simulink model "BESSINDPROJ"  (R2023b)
settings: Solver=VariableStepAuto  StartTime=0.0  StopTime=0.8  RelTol=1e-3
undefined symbols (not defined in the file): Ion, Lithium, Pnom1, Ts_Control, Ts_Power, Vnom_prim
libraries: spsSeriesRLCBranchLib x8, slpidlib x4, spsVoltageMeasurementLib x4, spsPowerLib x3, spsMeanLib x2, spsPWMGeneratorDCDCLib x2, spsCurrentMeasurementLib x2, spsMosfetLib x2, spsMultimeterLib x2, spsBatteryLib x1, spsSeriesRLCLoadLib x1, spsFundamentalPLLDrivenLib x1
settings Model: Creator=michelkhalil  LastModifiedBy=michelkhalil

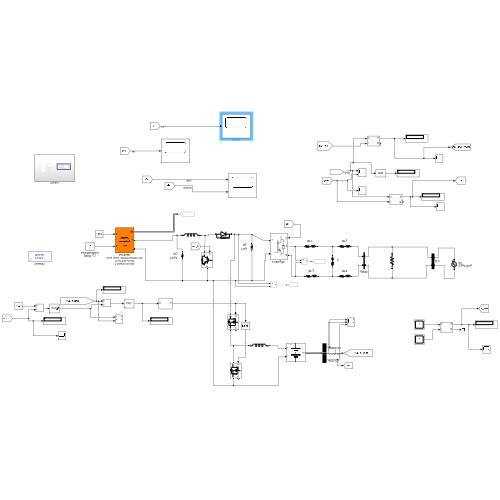
[thumbnail: Simulink's stored preview of the top-level diagram]
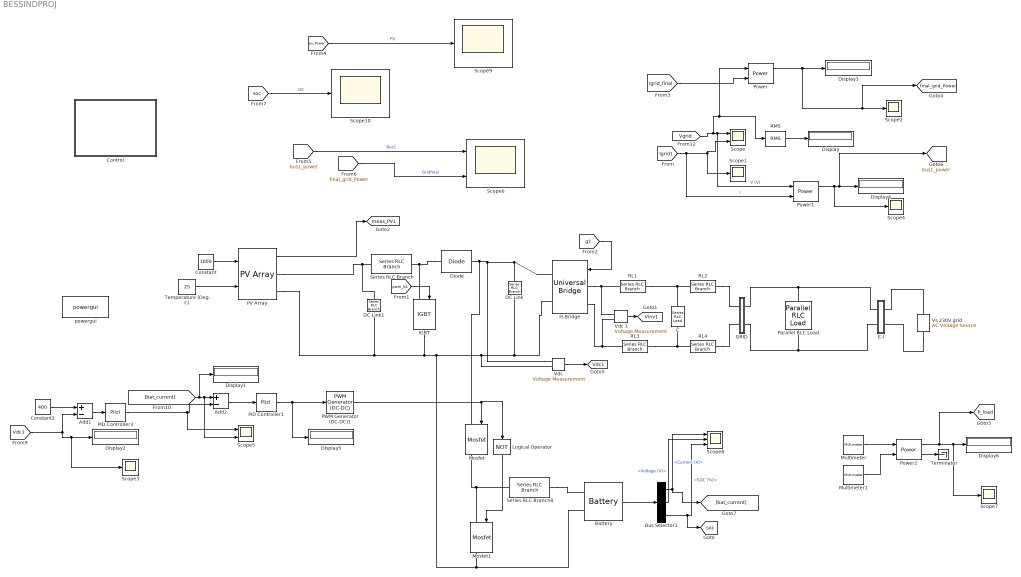
== system BESSINDPROJ ==
  Add1 : Sum  Inputs=+-
  Add2 : Sum  Inputs=+-
  Battery : spsBatteryLib/Battery  BatType=Lithium-Ion  ShowTempParam=off  ThermalPreset=no  ShowAgeParam=off  NomV=96  NomQ=50  SOC=60  Batt_Tr=30  PresetModel=on  MaxQ=50  MinV=72  FullV=111.7428  Dis_rate=21.7391  R=0.0192  Normal_OP=45.2174  expZone="[103.717      2.456522]"  current=[6.5 13 32.5]  Units=Time  Tci=20  NomT=20  T2=-30  MaxQ2=4.8  FullV2=7.1  Normal_OP2=5.655  expZone2="[6.58           1]"  Rca=0.6  ti=2000  Dp=0  Neq0=0  Tsim=1e6  Ta1=25  Qeol=5.4*0.9  Reol=0.013333*1.2  Char_age=[2.3478, 3]  Dis_age=[2.3478, 10]  N1=1500  N2=10500  N3=1000  N4=1400  Ta2=45  N5=950
  Bus Selector1 : BusSelector  OutputSignals=Current (A),Voltage (V),SOC (%)
  C : spsSeriesRLCLoadLib/Series RLC Load  LConnTagsString=a  RConnTagsString=__new0  NominalVoltage=240  NominalFrequency=50  ActivePower=10.5  InductivePower=0  CapacitivePower=525  Setx0=off  InitialVoltage=0  SetiL0=off  InitialCurrent=0  Measurements=None  LoadType=constant Z
  Constant : Constant  Value=1000
  Constant2 : Constant  Value=400
  Control : Subsystem
  DC Link : spsSeriesRLCBranchLib/Series RLC Branch  LConnTagsString=__new0  RConnTagsString=__new0  BranchType=C  Resistance=1.0  Inductance=1.0  SetiL0=off  InitialCurrent=0  Capacitance=3000e-6  Setx0=on  InitialVoltage=425  Measurements=None
  DC Link1 : spsSeriesRLCBranchLib/Series RLC Branch  LConnTagsString=__new0  RConnTagsString=__new0  BranchType=C  Resistance=1.0  Inductance=1.0  SetiL0=off  InitialCurrent=0  Capacitance=1000e-6  Setx0=on  InitialVoltage=260  Measurements=None
  Diode : spsDiodeLib/Diode  Ron=0.001  Lon=0  Vf=0.8  IC=0  UseSnubber=0  Rs=500  Cs=250e-9  Measurements=off
  Display{,1..6} (7 alike) : Display
  E-I : Subsystem
  GRID : Subsystem
  "H-Bridge " : spsUniversalBridgeLib/Universal Bridge  Arms=2  SnubberResistance=1e6  SnubberCapacitance=inf  Device=IGBT / Diodes  Ron=1e-3  Lon=0  ForwardVoltages=[ 0 0 ]  ForwardVoltage=0  GTOparameters=[ 10e-6 , 20e-6 ]  IGBTparameters=[ 1e-6 , 2e-6 ]*0  Measurements=None  Measurements_2=None  converterType=Rectifier
  IGBT : spsIGBTLib/IGBT  Ron=0.001  Lon=0  Vf=1  Tf=1e-6  Tt=2e-6  IC=0  Rs=1e5  Cs=inf  Measurements=off
  Logical Operator : Logic  Operator=NOT  AllPortsSameDT=off  OutDataTypeStr=boolean
  Mosfet : spsMosfetLib/Mosfet  Ron=0.1  Lon=0  Rd=0.01  Vfd=0  IC=0  Rs=1e6  Cs=inf  Measurements=on
  Mosfet1 : spsMosfetLib/Mosfet  Ron=0.1  Lon=0  Rd=0.01  Vfd=0  IC=0  Rs=1e6  Cs=inf  Measurements=on
  Multimeter : spsMultimeterLib/Multimeter  L=2  sel=1  yselected={}  Gain=1  OutputType=Complex  PlotAtSimulationStop=off  PhasorSimulation=off
  Multimeter1 : spsMultimeterLib/Multimeter  L=2  sel=2  yselected={}  Gain=1  OutputType=Complex  PlotAtSimulationStop=off  PhasorSimulation=off
  PID Controller1 : slpidlib/PID Controller  Controller=PI  Form=Parallel  TimeDomain=Discrete-time  UseExternalTs=off  SampleTime=Ts_Control  IntegratorMethod=Forward Euler  FilterMethod=Forward Euler  ControllerParametersSource=internal  P=7.90202765273144e-07  I=0.158040553054629  UseKiTs=off  D=0  N=100  UseFilter=on  TunerSelectOption=Transfer Function Based (PID Tuner App)  InitialConditionSource=internal  InitialConditionForIntegrator=0  InitialConditionForFilter=0  DifferentiatorICPrevScaledInput=0  ExternalReset=none  TrackingMode=off  Kt=1  LimitOutput=off  SatLimitsSource=internal  UpperSaturationLimit=inf  LowerSaturationLimit=-inf  LinearizeAsGain=on  AntiWindupMode=none  Kb=1  LimitIntegrator=off  UpperIntegratorSaturationLimit=inf  LowerIntegratorSaturationLimit=-inf  POutMin=[]  POutMax=[]  IOutMin=[]  IOutMax=[]  DOutMin=[]  DOutMax=[]  NOutMin=[]  NOutMax=[]  SumOutMin=[]  SumOutMax=[]  SaturationOutMin=[]  SaturationOutMax=[]  PParamMin=[]  PParamMax=[]  IParamMin=[]  IParamMax=[]  DParamMin=[]  DParamMax=[]  NParamMin=[]  NParamMax=[]  KbParamMin=[]  KbParamMax=[]  KtParamMin=[]  KtParamMax=[]  KbOutMin=[]  KbOutMax=[]  KtOutMin=[]  KtOutMax=[]  IntegratorOutMin=[]  IntegratorOutMax=[]  FilterOutMin=[]  FilterOutMax=[]  SumI1OutMin=[]  SumI1OutMax=[]  SumI2OutMin=[]  SumI2OutMax=[]  SumI3OutMin=[]  SumI3OutMax=[]  SumI4OutMin=[]  SumI4OutMax=[]  SumDOutMin=[]  SumDOutMax=[]  DifferentiatorOutMin=[]  DifferentiatorOutMax=[]  FilterDiffOutCoefMin=[]  FilterDiffOutCoefMax=[]  ReciprocalOutMin=[]  ReciprocalOutMax=[]  SumDenOutMin=[]  SumDenOutMax=[]  SumNumOutMin=[]  SumNumOutMax=[]  DivideOutMin=[]  DivideOutMax=[]  UdiffTsProdOutMin=[]  UdiffTsProdOutMax=[]  NTsProdOutMin=[]  NTsProdOutMax=[]  UintegralTsProdOutMin=[]  UintegralTsProdOutMax=[]  UngainTsProdOutMin=[]  UngainTsProdOutMax=[]  ClampingZeroOutDataTypeStr=Inherit: Inherit via back propagation  ClampingZeroOutMin=[]  ClampingZeroOutMax=[]  FilterDenConstantOutDataTypeStr=Inherit: Inherit via back propagation  FilterDenConstantOutMin=[]  FilterDenConstantOutMax=[]  PCopyOutDataTypeStr=Inherit: Inherit via back propagation  PCopyOutMin=[]  PCopyOutMax=[]  NCopyOutDataTypeStr=Inherit: Inherit via back propagation  NCopyOutMin=[]  NCopyOutMax=[]  IntegratorContinuousStateAttributes=''  IntegratorStateMustResolveToSignalObject=off  IntegratorRTWStateStorageClass=Auto  FilterContinuousStateAttributes=''  FilterStateMustResolveToSignalObject=off  FilterRTWStateStorageClass=Auto  ParallelPVariant=InternalParameters  IdealPVariant=Disabled  IVariant=InternalParameters  DVariant=Disabled  IntegratorVariant=Discrete  SatVariant=Disabled  AWVariant=Passthrough  PCopyVariant=Disabled  TRVariant=Disabled  FdbkBlocksVariant=Forward  IdealPFdbkVariant=Disabled  SatFdbkVariant=Disabled  DerivativeFilterVariant=Disabled  NVariant=Disabled  NCopyVariant=Disabled_SignalSpec  FilterICVariant=Disabled  IntegratorICVariant=InternalICs  ExternalResetVariant=Disabled  TRSumVariant=Passthrough  SumFdbkVariant=Disabled  SumVariant=Sum_PI  TsampFilterVariant=InternalTs  TsampNgainVariant=Passthrough  TsampIntegralVariant=Disabled_SignalSpec  ExternalSaturationOutDataTypeStr=Inherit: Same as second input
  PID Controller3 : slpidlib/PID Controller  Controller=PI  Form=Parallel  TimeDomain=Discrete-time  UseExternalTs=off  SampleTime=Ts_Control*20  IntegratorMethod=Forward Euler  FilterMethod=Forward Euler  ControllerParametersSource=internal  P=0.557452904708  I=9.2264574519469  UseKiTs=off  D=0  N=100  UseFilter=on  TunerSelectOption=Transfer Function Based (PID Tuner App)  InitialConditionSource=internal  InitialConditionForIntegrator=0  InitialConditionForFilter=0  DifferentiatorICPrevScaledInput=0  ExternalReset=none  TrackingMode=off  Kt=1  LimitOutput=on  SatLimitsSource=internal  UpperSaturationLimit=120  LowerSaturationLimit=-120  LinearizeAsGain=on  AntiWindupMode=none  Kb=1  LimitIntegrator=off  UpperIntegratorSaturationLimit=inf  LowerIntegratorSaturationLimit=-inf  POutMin=[]  POutMax=[]  IOutMin=[]  IOutMax=[]  DOutMin=[]  DOutMax=[]  NOutMin=[]  NOutMax=[]  SumOutMin=[]  SumOutMax=[]  SaturationOutMin=[]  SaturationOutMax=[]  PParamMin=[]  PParamMax=[]  IParamMin=[]  IParamMax=[]  DParamMin=[]  DParamMax=[]  NParamMin=[]  NParamMax=[]  KbParamMin=[]  KbParamMax=[]  KtParamMin=[]  KtParamMax=[]  KbOutMin=[]  KbOutMax=[]  KtOutMin=[]  KtOutMax=[]  IntegratorOutMin=[]  IntegratorOutMax=[]  FilterOutMin=[]  FilterOutMax=[]  SumI1OutMin=[]  SumI1OutMax=[]  SumI2OutMin=[]  SumI2OutMax=[]  SumI3OutMin=[]  SumI3OutMax=[]  SumI4OutMin=[]  SumI4OutMax=[]  SumDOutMin=[]  SumDOutMax=[]  DifferentiatorOutMin=[]  DifferentiatorOutMax=[]  FilterDiffOutCoefMin=[]  FilterDiffOutCoefMax=[]  ReciprocalOutMin=[]  ReciprocalOutMax=[]  SumDenOutMin=[]  SumDenOutMax=[]  SumNumOutMin=[]  SumNumOutMax=[]  DivideOutMin=[]  DivideOutMax=[]  UdiffTsProdOutMin=[]  UdiffTsProdOutMax=[]  NTsProdOutMin=[]  NTsProdOutMax=[]  UintegralTsProdOutMin=[]  UintegralTsProdOutMax=[]  UngainTsProdOutMin=[]  UngainTsProdOutMax=[]  ClampingZeroOutDataTypeStr=Inherit: Inherit via back propagation  ClampingZeroOutMin=[]  ClampingZeroOutMax=[]  FilterDenConstantOutDataTypeStr=Inherit: Inherit via back propagation  FilterDenConstantOutMin=[]  FilterDenConstantOutMax=[]  PCopyOutDataTypeStr=Inherit: Inherit via back propagation  PCopyOutMin=[]  PCopyOutMax=[]  NCopyOutDataTypeStr=Inherit: Inherit via back propagation  NCopyOutMin=[]  NCopyOutMax=[]  IntegratorContinuousStateAttributes=''  IntegratorStateMustResolveToSignalObject=off  IntegratorRTWStateStorageClass=Auto  FilterContinuousStateAttributes=''  FilterStateMustResolveToSignalObject=off  FilterRTWStateStorageClass=Auto  ParallelPVariant=InternalParameters  IdealPVariant=Disabled  IVariant=InternalParameters  DVariant=Disabled  IntegratorVariant=Discrete  SatVariant=Enabled  AWVariant=Passthrough  PCopyVariant=Disabled  TRVariant=Disabled  FdbkBlocksVariant=Forward  IdealPFdbkVariant=Disabled  SatFdbkVariant=Disabled  DerivativeFilterVariant=Disabled  NVariant=Disabled  NCopyVariant=Disabled_SignalSpec  FilterICVariant=Disabled  IntegratorICVariant=InternalICs  ExternalResetVariant=Disabled  TRSumVariant=Passthrough  SumFdbkVariant=Disabled  SumVariant=Sum_PI  TsampFilterVariant=InternalTs  TsampNgainVariant=Passthrough  TsampIntegralVariant=Disabled_SignalSpec  ExternalSaturationOutDataTypeStr=Inherit: Same as second input
  PV Array : spsPVArrayLib/PV Array  Npar=2  Nser=9  PlotType=array @ 25 deg.C & specified irradiances  S_vec="[ 1000  750 500  250 ]"  Temp_C_vec=[ 45 25 100 ]  ModuleName=Trina Solar TSM-225PA05.xy2  PlotWhenSelected=off  Pm=225.204  Ncell=60  Voc=36.9  Isc=8.2  Vm=29.4  Im=7.66  beta_Voc_pc=-0.31  alpha_Isc_pc=0.05  beta_Voc=-0.11439  alpha_Isc=0.0041  IL=8.2156  I0=4.2072e-11  nI=0.92146  Rsh=224.5497  Rs=0.42703  RobustModel=off  RobustCellTemperature=25  BAL=on  Tc=1e-6  Tfilter=5e-5
      settings: AttributesFormatString=|
      | %<ModuleName>
      | %<Nser>-module string
      | %<Npar> parallel strings
  PWM Generator (DC-DC)1 : spsPWMGeneratorDCDCLib/PWM Generator (DC-DC)  Fsw=5000  Ts=Ts_Power
  Parallel RLC Load : spsParallelRLCLoadLib/Parallel RLC Load  LConnTagsString=a  RConnTagsString=__new0  NominalVoltage=230  NominalFrequency=50  ActivePower=3e3  InductivePower=0  CapacitivePower=0  Setx0=off  InitialVoltage=0  SetiL0=off  InitialCurrent=0  Measurements=Branch voltage and current  LoadType=constant Z
      settings: AttributesFormatString=\n  LibrarySourceBlock=sps_lib/Passives/Parallel RLC Load
  Power : spsPowerLib/Power  Freq=50  Vinit=[1, 0]  Iinit=[1, 0]  Ts=0
  Power1 : spsPowerLib/Power  Freq=50  Vinit=[1, 0]  Iinit=[1, 0]  Ts=0
  Power2 : spsPowerLib/Power  Freq=50  Vinit=[1, 0]  Iinit=[1, 0]  Ts=0
  RL{1..4} (4 alike) : spsSeriesRLCBranchLib/Series RLC Branch  LConnTagsString=__new0  RConnTagsString=__new0  BranchType=RL  Resistance=8.23e-3  Inductance=2.183e-3  SetiL0=off  InitialCurrent=0  Capacitance=1e-6  Setx0=off  InitialVoltage=0  Measurements=None
  RMS : spsRMSLib/RMS  TrueRMS=on  Freq=50  RMSInit=230  Ts=Ts_Power
  Scope : Scope  NumInputPorts=2
  Scope{1..4,7,9..10} (7 alike) : Scope
  Scope5 : Scope  NumInputPorts=2
  Scope6 : Scope  NumInputPorts=2
  Scope8 : Scope  NumInputPorts=3
  Series RLC Branch : spsSeriesRLCBranchLib/Series RLC Branch  LConnTagsString=__new0  RConnTagsString=__new0  BranchType=L  Resistance=1  Inductance=3e-3  SetiL0=off  InitialCurrent=0  Capacitance=1e-6  Setx0=off  InitialVoltage=0  Measurements=None
  Series RLC Branch8 : spsSeriesRLCBranchLib/Series RLC Branch  LConnTagsString=__new0  RConnTagsString=__new0  BranchType=L  Resistance=1  Inductance=1e-3  SetiL0=off  InitialCurrent=0  Capacitance=1e-6  Setx0=off  InitialVoltage=0  Measurements=None
  Temperature (Deg. C) : Constant  Value=25
  Terminator : Terminator
  "Vdc " : spsVoltageMeasurementLib/Voltage Measurement  Tag=PoWeRsYsTeMmEaSuReMeNt  PhasorSimulation=off  OutputType=Magnitude  PSBequivalent=0
  Vdc 1 : spsVoltageMeasurementLib/Voltage Measurement  Tag=PoWeRsYsTeMmEaSuReMeNt  PhasorSimulation=off  OutputType=Magnitude  PSBequivalent=0
  Vs 230V grid : spsACVoltageSourceLib/AC Voltage Source  Description=source block  Amplitude=230*sqrt(2)  Phase=0  Frequency=50  SampleTime=0  Measurements=None  BusType=swing  Pref=10e3  Qref=0  Qmin=-inf  Qmax=+inf
      settings: AttributesFormatString=\n
  powergui : sps_lib/powergui  Priority=1  SimulationMode=Discrete  SampleTime=Ts_Power  frequency=60  Iterations=50  frequencyindice=0  Pbase=100e6  ErrMax=1e-4  UnitsV=kV  UnitsW=MW  buscounter=0  FunctionMessages=off  echomessages=off  EnableUseOfTLC=off  CurrentSourceSwitches=off  DisableSnubberDevices=off  DisableRonSwitches=off  DisableVfSwitches=off  DisplayEquations=off  AutomaticDiscreteSolvers=off  SolverType=Tustin/Backward Euler (TBE)  Interpol=off  ExternalGateDelay=off  methode=off  Ts=0  x0status=blocks  SPID=off  SwTol=0  HookPort=off  NonlinearTolerance=1e-8  nMaxIteration=5  ContinueOnMaxIteration=on  RestoreLinks=warning  ResistiveCurrentMeasurement=off  Frange=[0:2:500]  Ylog=off  Xlog=on  ShowGrid=off  save=off  variable=ZData  structure=VIgrid  ZoomFFT=off  StartTime=0.55  cycles=1  DisplayStyle=1  fundamental=60  FreqAxis=on  MaxFrequency=10000  frequencyindicesteady=1  RmsSteady=1  display=off
  tag scope: P_load=global, Vdc1=global, Vinv1=global, bus1_power=global, final_grid_Power=global, meas_PV1=global, soc=global
  wires:
  RMS/1 -> Display/1
  Multimeter1/1 -> Power2/2
  [final_grid_Power] -> Scope6/2  "Gridfinal"
  [Vdc1] -> Scope3/1, Display2/1, Add1/2
  Constant2/1 -> Add1/1
  Bus Selector1/1 -> [bat_current], Scope8/1  "<Current (A)>"
  Power2/1 -> [P_load], Scope7/1, Display6/1
  Battery/1 -> Bus Selector1/1
  Add1/1 -> PID Controller3/1
  Temperature (Deg. C)/1 -> PV Array/2
  PWM Generator (DC-DC)1/1 -> Logical Operator/1, Mosfet/1
  PID Controller1/1 -> Display5/1, PWM Generator (DC-DC)1/1
  Bus Selector1/3 -> [soc], Scope8/3  "<SOC (%)>"
  Power/1 -> [final_grid_Power], Scope2/1, Display3/1
  [pwm_b1] -> IGBT/1
  [Igrid_final] -> Power/2
  Add2/1 -> PID Controller1/1
  Constant/1 -> PV Array/1
  Logical Operator/1 -> Mosfet1/1
  [bat_current] -> Scope5/2, Add2/1, Display1/1
  PID Controller3/1 -> Scope5/1, Add2/2
  [g1] -> "H-Bridge "/1
  Vdc 1/1 -> [Vinv1]
  Bus Selector1/2 -> Scope8/2  "<Voltage (V)>"
  [bus1_power] -> Scope6/1  "Bus1"
  [Vgrid] -> Power/1, RMS/1, Power1/1, Scope/1  "V (V)"
  Power2/2 -> Terminator/1
  PV Array/1 -> [meas_PV1]
  "Vdc "/1 -> [Vdc1]
  Multimeter/1 -> Power2/1
  [Igrid1] -> Power1/2, Scope/2, Scope1/1  "I"
  Power1/1 -> Scope4/1, [bus1_power], Display4/1
  [pv_Power] -> Scope9/1  "PV"
  [soc] -> Scope10/1  "soc"
  connections:
  "H-Bridge "/LConn2 -- RL3/LConn1 -- Vdc 1/LConn2
  IGBT/RConn1 -- PV Array/RConn2 -- DC Link1/RConn1 -- DC Link/RConn1 -- "H-Bridge "/RConn2 -- "Vdc "/LConn2 -- Mosfet1/RConn1 -- Battery/LConn2
  "Vdc "/LConn1 -- DC Link/LConn1 -- "H-Bridge "/RConn1 -- Diode/RConn1 -- Mosfet/LConn1
  Parallel RLC Load/RConn1 -- E-I/LConn2 -- GRID/RConn2
  Mosfet/RConn1 -- Series RLC Branch8/LConn1 -- Mosfet1/LConn1
  "H-Bridge "/LConn1 -- Vdc 1/LConn1 -- RL1/LConn1
  RL1/RConn1 -- RL2/LConn1 -- C/RConn1
  Diode/LConn1 -- Series RLC Branch/RConn1 -- IGBT/LConn1
  Series RLC Branch/LConn1 -- PV Array/RConn1 -- DC Link1/LConn1
  Parallel RLC Load/LConn1 -- E-I/LConn1 -- GRID/RConn1
  RL3/RConn1 -- C/LConn1 -- RL4/LConn1
  Series RLC Branch8/RConn1 -- Battery/LConn1
  Vs 230V grid/LConn1 -- E-I/RConn2
  RL2/RConn1 -- GRID/LConn1
  Vs 230V grid/RConn1 -- E-I/RConn1
  RL4/RConn1 -- GRID/LConn2

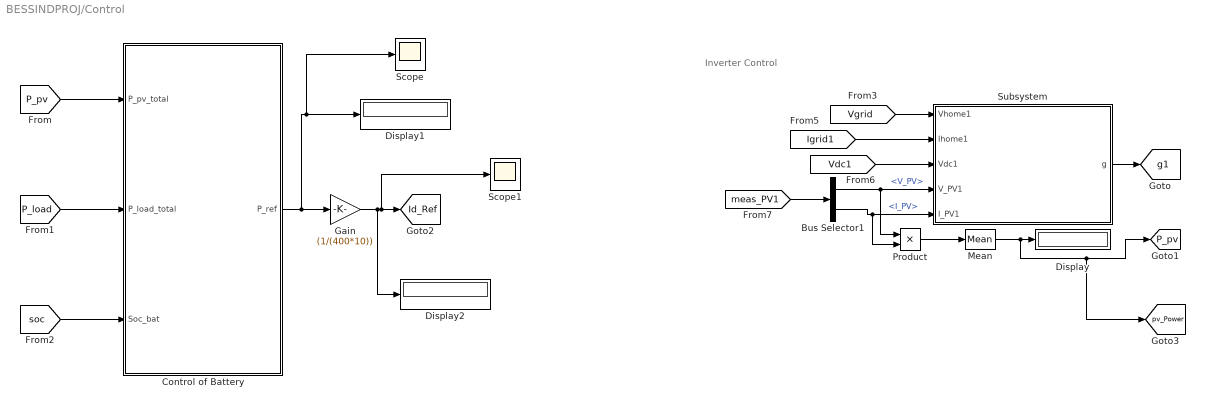
== system BESSINDPROJ/Control ==
  note: Inverter Control
  Bus Selector1 : BusSelector  OutputSignals=V_PV,I_PV
  Control of Battery : Stateflow chart  TreatAsAtomicUnit=on
  Display : Display
  Display1 : Display
  Display2 : Display
  Gain : Gain  Gain=(1/(400*10))
  Mean : spsMeanLib/Mean  Freq=50  Vinit=0  Ts=0
  Product : Product
  Scope : Scope
  Scope1 : Scope
  Subsystem : Subsystem
  tag scope: Id_Ref=global, P_pv=global, g1=global, pv_Power=global
  wires:
  Bus Selector1/1 -> Product/1, Subsystem/4(V_PV1)  "<V_PV>"
  Bus Selector1/2 -> Product/2, Subsystem/5(I_PV1)  "<I_PV>"
  [meas_PV1] -> Bus Selector1/1
  Subsystem/1(g) -> [g1]
  [Vgrid] -> Subsystem/1(Vhome1)
  [Igrid1] -> Subsystem/2(Ihome1)
  [Vdc1] -> Subsystem/3(Vdc1)
  Product/1 -> Mean/1
  Mean/1 -> [pv_Power], [P_pv], Display/1
  [P_pv] -> Control of Battery/1(P_pv_total)
  [P_load] -> Control of Battery/2(P_load_total)
  [soc] -> Control of Battery/3(Soc_bat)
  Control of Battery/1(P_ref) -> Scope/1, Display1/1, Gain/1
  Gain/1 -> Display2/1, Scope1/1, [Id_Ref]

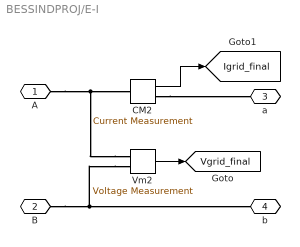
== system BESSINDPROJ/E-I ==
  CM2 : spsCurrentMeasurementLib/Current Measurement  PhasorSimulation=off  OutputType=Complex  PSBequivalent=0
  Vm2 : spsVoltageMeasurementLib/Voltage Measurement  PhasorSimulation=off  OutputType=Complex  PSBequivalent=0
  A : PMIOPort  Side=Left
  B : PMIOPort  Port=2  Side=Left
  a : PMIOPort  Port=3  Side=Right
  b : PMIOPort  Port=4  Side=Right
  tag scope: Igrid_final=global, Vgrid_final=global
  wires:
  Vm2/1 -> [Vgrid_final]
  CM2/1 -> [Igrid_final]
  connections:
  Vm2/LConn2 -- b/RConn1 -- B/RConn1
  Vm2/LConn1 -- A/RConn1 -- CM2/LConn1
  CM2/RConn1 -- a/RConn1

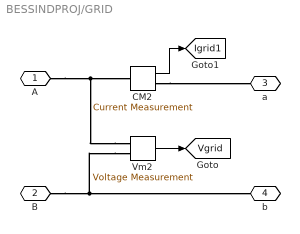
== system BESSINDPROJ/GRID ==
  CM2 : spsCurrentMeasurementLib/Current Measurement  PhasorSimulation=off  OutputType=Complex  PSBequivalent=0
  Vm2 : spsVoltageMeasurementLib/Voltage Measurement  PhasorSimulation=off  OutputType=Complex  PSBequivalent=0
  A : PMIOPort  Side=Left
  B : PMIOPort  Port=2  Side=Left
  a : PMIOPort  Port=3  Side=Right
  b : PMIOPort  Port=4  Side=Right
  tag scope: Igrid1=global, Vgrid=global
  wires:
  Vm2/1 -> [Vgrid]
  CM2/1 -> [Igrid1]
  connections:
  Vm2/LConn2 -- b/RConn1 -- B/RConn1
  Vm2/LConn1 -- A/RConn1 -- CM2/LConn1
  CM2/RConn1 -- a/RConn1

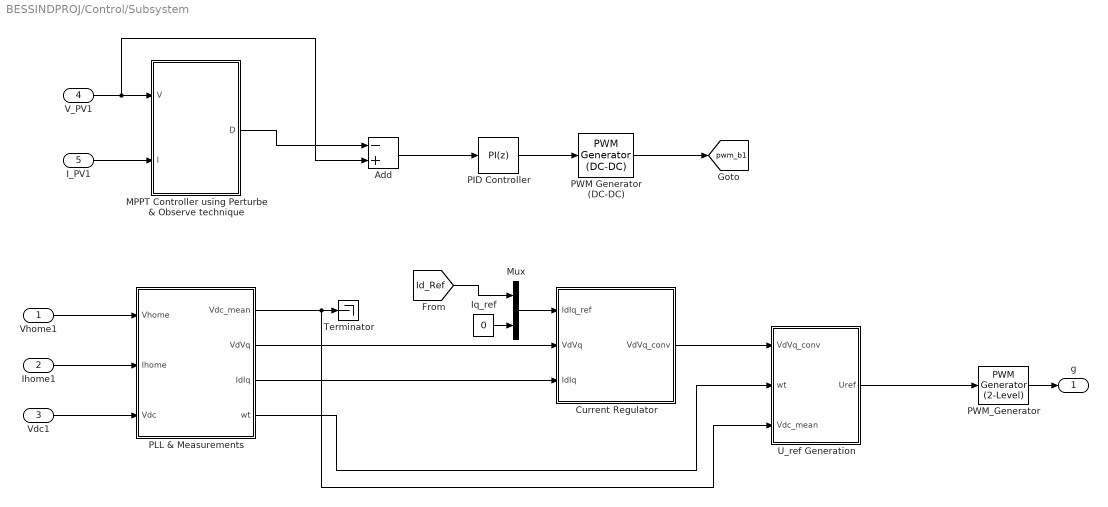
== system BESSINDPROJ/Control/Subsystem ==
  Vhome1 : Inport  PortDimensions=1
  Ihome1 : Inport  Port=2  PortDimensions=1
  Vdc1 : Inport  Port=3  PortDimensions=1
  V_PV1 : Inport  Port=4  PortDimensions=1
  I_PV1 : Inport  Port=5  PortDimensions=1
  Add : Sum  Inputs=-+
  Current Regulator : Subsystem
  Iq_ref : Constant  Value=0
  "MPPT Controller using Perturbe & Observe technique " : MATLAB Function  TreatAsAtomicUnit=on
  Mux : Mux  Inputs=2
  PID Controller : slpidlib/PID Controller  Controller=PI  Form=Parallel  TimeDomain=Discrete-time  UseExternalTs=off  SampleTime=Ts_Control  IntegratorMethod=Forward Euler  FilterMethod=Forward Euler  ControllerParametersSource=internal  P=1.3250761095226e-06  I=0.26501522190452  UseKiTs=off  D=0  N=100  UseFilter=on  TunerSelectOption=Transfer Function Based (PID Tuner App)  InitialConditionSource=internal  InitialConditionForIntegrator=0  InitialConditionForFilter=0  DifferentiatorICPrevScaledInput=0  ExternalReset=none  TrackingMode=off  Kt=1  LimitOutput=off  SatLimitsSource=internal  UpperSaturationLimit=inf  LowerSaturationLimit=-inf  LinearizeAsGain=on  AntiWindupMode=none  Kb=1  LimitIntegrator=off  UpperIntegratorSaturationLimit=inf  LowerIntegratorSaturationLimit=-inf  POutMin=[]  POutMax=[]  IOutMin=[]  IOutMax=[]  DOutMin=[]  DOutMax=[]  NOutMin=[]  NOutMax=[]  SumOutMin=[]  SumOutMax=[]  SaturationOutMin=[]  SaturationOutMax=[]  PParamMin=[]  PParamMax=[]  IParamMin=[]  IParamMax=[]  DParamMin=[]  DParamMax=[]  NParamMin=[]  NParamMax=[]  KbParamMin=[]  KbParamMax=[]  KtParamMin=[]  KtParamMax=[]  KbOutMin=[]  KbOutMax=[]  KtOutMin=[]  KtOutMax=[]  IntegratorOutMin=[]  IntegratorOutMax=[]  FilterOutMin=[]  FilterOutMax=[]  SumI1OutMin=[]  SumI1OutMax=[]  SumI2OutMin=[]  SumI2OutMax=[]  SumI3OutMin=[]  SumI3OutMax=[]  SumI4OutMin=[]  SumI4OutMax=[]  SumDOutMin=[]  SumDOutMax=[]  DifferentiatorOutMin=[]  DifferentiatorOutMax=[]  FilterDiffOutCoefMin=[]  FilterDiffOutCoefMax=[]  ReciprocalOutMin=[]  ReciprocalOutMax=[]  SumDenOutMin=[]  SumDenOutMax=[]  SumNumOutMin=[]  SumNumOutMax=[]  DivideOutMin=[]  DivideOutMax=[]  UdiffTsProdOutMin=[]  UdiffTsProdOutMax=[]  NTsProdOutMin=[]  NTsProdOutMax=[]  UintegralTsProdOutMin=[]  UintegralTsProdOutMax=[]  UngainTsProdOutMin=[]  UngainTsProdOutMax=[]  ClampingZeroOutDataTypeStr=Inherit: Inherit via back propagation  ClampingZeroOutMin=[]  ClampingZeroOutMax=[]  FilterDenConstantOutDataTypeStr=Inherit: Inherit via back propagation  FilterDenConstantOutMin=[]  FilterDenConstantOutMax=[]  PCopyOutDataTypeStr=Inherit: Inherit via back propagation  PCopyOutMin=[]  PCopyOutMax=[]  NCopyOutDataTypeStr=Inherit: Inherit via back propagation  NCopyOutMin=[]  NCopyOutMax=[]  IntegratorContinuousStateAttributes=''  IntegratorStateMustResolveToSignalObject=off  IntegratorRTWStateStorageClass=Auto  FilterContinuousStateAttributes=''  FilterStateMustResolveToSignalObject=off  FilterRTWStateStorageClass=Auto  ParallelPVariant=InternalParameters  IdealPVariant=Disabled  IVariant=InternalParameters  DVariant=Disabled  IntegratorVariant=Discrete  SatVariant=Disabled  AWVariant=Passthrough  PCopyVariant=Disabled  TRVariant=Disabled  FdbkBlocksVariant=Forward  IdealPFdbkVariant=Disabled  SatFdbkVariant=Disabled  DerivativeFilterVariant=Disabled  NVariant=Disabled  NCopyVariant=Disabled_SignalSpec  FilterICVariant=Disabled  IntegratorICVariant=InternalICs  ExternalResetVariant=Disabled  TRSumVariant=Passthrough  SumFdbkVariant=Disabled  SumVariant=Sum_PI  TsampFilterVariant=InternalTs  TsampNgainVariant=Passthrough  TsampIntegralVariant=Disabled_SignalSpec  ExternalSaturationOutDataTypeStr=Inherit: Same as second input
  PLL & Measurements : Subsystem
  PWM Generator (DC-DC) : spsPWMGeneratorDCDCLib/PWM Generator (DC-DC)  Fsw=10e3  Ts=Ts_Control
  PWM_Generator : spsPWMGenerator2LevelLib/PWM Generator (2-Level)  ModulatorType=Single-phase full-bridge - Bipolar modulation (4 pulses)  ModulatorMode=Unsynchronized  Fc=5e3  Pc=90  nF=27  MinMax="[ -1  1 ]"  SamplingTechnique=Asymmetrical regular (double edge)  ModulatingSignals=off  m=0.8  Freq=60  Phase=0  Ts=Ts_Power  ShowCarrierOutport=off
      settings: AttributesFormatString=%<ModulatorType>
  Terminator : Terminator
  "U_ref Generation " : Subsystem
  g : Outport  VectorParamsAs1DForOutWhenUnconnected=off
  tag scope: pwm_b1=global
  wires:
  Ihome1/1 -> PLL & Measurements/2(Ihome)
  "MPPT Controller using Perturbe & Observe technique "/1(D) -> Add/1
  PID Controller/1 -> PWM Generator (DC-DC)/1
  "U_ref Generation "/1(Uref) -> PWM_Generator/1
  PLL & Measurements/2(VdVq) -> Current Regulator/2(VdVq)
  PLL & Measurements/4(wt) -> "U_ref Generation "/2(wt)
  Current Regulator/1(VdVq_conv) -> "U_ref Generation "/1(VdVq_conv)
  PLL & Measurements/3(IdIq) -> Current Regulator/3(IdIq)
  PWM Generator (DC-DC)/1 -> [pwm_b1]
  PWM_Generator/1 -> g/1
  Add/1 -> PID Controller/1
  Vdc1/1 -> PLL & Measurements/3(Vdc)
  Iq_ref/1 -> Mux/2
  V_PV1/1 -> Add/2, "MPPT Controller using Perturbe & Observe technique "/1(V)
  PLL & Measurements/1(Vdc_mean) -> Terminator/1, "U_ref Generation "/3(Vdc_mean)
  Mux/1 -> Current Regulator/1(IdIq_ref)
  I_PV1/1 -> "MPPT Controller using Perturbe & Observe technique "/2(I)
  Vhome1/1 -> PLL & Measurements/1(Vhome)
  [Id_Ref] -> Mux/1

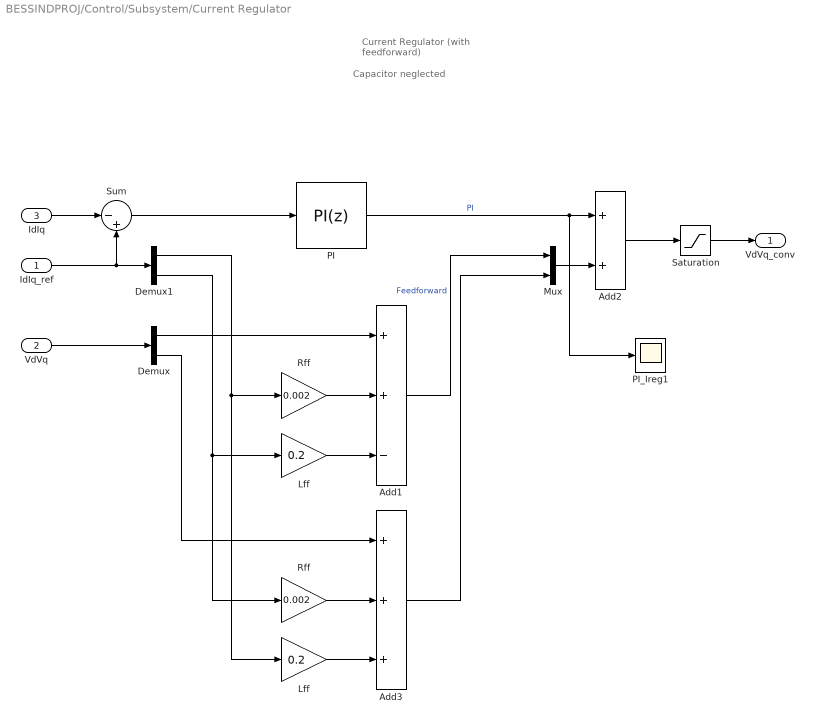
== system BESSINDPROJ/Control/Subsystem/Current Regulator ==
  note: Current Regulator
      | (with feedforward)
  note: Capacitor neglected
  IdIq_ref : Inport  PortDimensions=2
  VdVq : Inport  Port=2  PortDimensions=2
  IdIq : Inport  Port=3  PortDimensions=2
  Add1 : Sum  Inputs=++-
  Add2 : Sum
  Add3 : Sum  Inputs=+++
  Demux : Demux  Outputs=2
  Demux1 : Demux  Outputs=2
  Lff : Gain  Gain=0.2  SaturateOnIntegerOverflow=on  OutDataTypeStr=Inherit: Same as input  ParamDataTypeStr=Inherit: Same as input
  "Lff  " : Gain  Gain=0.2  SaturateOnIntegerOverflow=on  OutDataTypeStr=Inherit: Same as input  ParamDataTypeStr=Inherit: Same as input
  Mux : Mux  Inputs=2
  PI : slpidlib/PID Controller  Controller=PI  Form=Parallel  TimeDomain=Discrete-time  UseExternalTs=off  SampleTime=Ts_Control  IntegratorMethod=Forward Euler  FilterMethod=Forward Euler  ControllerParametersSource=internal  P=0.15  I=6.6  UseKiTs=off  D=0  N=100  UseFilter=on  TunerSelectOption=Transfer Function Based (PID Tuner App)  InitialConditionSource=internal  InitialConditionForIntegrator=0  InitialConditionForFilter=0  DifferentiatorICPrevScaledInput=0  ExternalReset=none  TrackingMode=off  Kt=1  LimitOutput=on  SatLimitsSource=internal  UpperSaturationLimit=1.5  LowerSaturationLimit=-1.5  LinearizeAsGain=off  AntiWindupMode=none  Kb=1  LimitIntegrator=off  UpperIntegratorSaturationLimit=inf  LowerIntegratorSaturationLimit=-inf  POutMin=[]  POutMax=[]  IOutMin=[]  IOutMax=[]  DOutMin=[]  DOutMax=[]  NOutMin=[]  NOutMax=[]  SumOutMin=[]  SumOutMax=[]  SaturationOutMin=[]  SaturationOutMax=[]  PParamMin=[]  PParamMax=[]  IParamMin=[]  IParamMax=[]  DParamMin=[]  DParamMax=[]  NParamMin=[]  NParamMax=[]  KbParamMin=[]  KbParamMax=[]  KtParamMin=[]  KtParamMax=[]  KbOutMin=[]  KbOutMax=[]  KtOutMin=[]  KtOutMax=[]  IntegratorOutMin=[]  IntegratorOutMax=[]  FilterOutMin=[]  FilterOutMax=[]  SumI1OutMin=[]  SumI1OutMax=[]  SumI2OutMin=[]  SumI2OutMax=[]  SumI3OutMin=[]  SumI3OutMax=[]  SumI4OutMin=[]  SumI4OutMax=[]  SumDOutMin=[]  SumDOutMax=[]  DifferentiatorOutMin=[]  DifferentiatorOutMax=[]  FilterDiffOutCoefMin=[]  FilterDiffOutCoefMax=[]  ReciprocalOutMin=[]  ReciprocalOutMax=[]  SumDenOutMin=[]  SumDenOutMax=[]  SumNumOutMin=[]  SumNumOutMax=[]  DivideOutMin=[]  DivideOutMax=[]  UdiffTsProdOutMin=[]  UdiffTsProdOutMax=[]  NTsProdOutMin=[]  NTsProdOutMax=[]  UintegralTsProdOutMin=[]  UintegralTsProdOutMax=[]  UngainTsProdOutMin=[]  UngainTsProdOutMax=[]  ClampingZeroOutDataTypeStr=Inherit: Inherit via back propagation  ClampingZeroOutMin=[]  ClampingZeroOutMax=[]  FilterDenConstantOutDataTypeStr=Inherit: Inherit via back propagation  FilterDenConstantOutMin=[]  FilterDenConstantOutMax=[]  PCopyOutDataTypeStr=Inherit: Inherit via back propagation  PCopyOutMin=[]  PCopyOutMax=[]  NCopyOutDataTypeStr=Inherit: Inherit via back propagation  NCopyOutMin=[]  NCopyOutMax=[]  IntegratorContinuousStateAttributes=''  IntegratorStateMustResolveToSignalObject=off  IntegratorRTWStateStorageClass=Auto  FilterContinuousStateAttributes=''  FilterStateMustResolveToSignalObject=off  FilterRTWStateStorageClass=Auto  ParallelPVariant=InternalParameters  IdealPVariant=Disabled  IVariant=InternalParameters  DVariant=Disabled  IntegratorVariant=Discrete  SatVariant=Enabled  AWVariant=Passthrough  PCopyVariant=Disabled  TRVariant=Disabled  FdbkBlocksVariant=Forward  IdealPFdbkVariant=Disabled  SatFdbkVariant=Disabled  DerivativeFilterVariant=Disabled  NVariant=Disabled  NCopyVariant=Disabled_SignalSpec  FilterICVariant=Disabled  IntegratorICVariant=InternalICs  ExternalResetVariant=Disabled  TRSumVariant=Passthrough  SumFdbkVariant=Disabled  SumVariant=Sum_PI  TsampFilterVariant=InternalTs  TsampNgainVariant=Passthrough  TsampIntegralVariant=Disabled_SignalSpec  ExternalSaturationOutDataTypeStr=Inherit: Same as second input
  PI_Ireg1 : Scope
  Rff : Gain  Gain=0.002  SaturateOnIntegerOverflow=on  OutDataTypeStr=Inherit: Same as input  ParamDataTypeStr=Inherit: Same as input
  "Rff " : Gain  Gain=0.002  SaturateOnIntegerOverflow=on  OutDataTypeStr=Inherit: Same as input  ParamDataTypeStr=Inherit: Same as input
  Saturation : Saturate  UpperLimit=1.5  LowerLimit=-1.5
  Sum : Sum  Inputs=|-+
  VdVq_conv : Outport  VectorParamsAs1DForOutWhenUnconnected=off
  wires:
  Add3/1 -> Mux/2
  Demux/2 -> Add3/1
  Add1/1 -> Mux/1  "Feedforward"
  Lff/1 -> Add3/3
  Rff/1 -> Add3/2
  Demux1/2 -> Rff/1, "Lff  "/1
  "Lff  "/1 -> Add1/3
  Demux1/1 -> Lff/1, "Rff "/1
  "Rff "/1 -> Add1/2
  Demux/1 -> Add1/1
  VdVq/1 -> Demux/1
  Saturation/1 -> VdVq_conv/1
  Add2/1 -> Saturation/1
  IdIq/1 -> Sum/1
  IdIq_ref/1 -> Demux1/1, Sum/2
  Sum/1 -> PI/1
  PI/1 -> Add2/1, PI_Ireg1/1  "PI"
  Mux/1 -> Add2/2

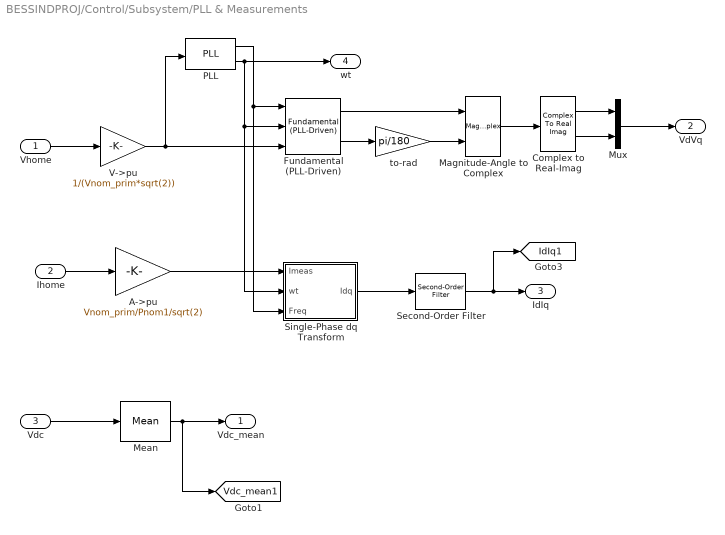
== system BESSINDPROJ/Control/Subsystem/PLL & Measurements ==
  Vhome : Inport
  Ihome : Inport  Port=2
  Vdc : Inport  Port=3
  A->pu : Gain  Gain=Vnom_prim/Pnom1/sqrt(2)  SaturateOnIntegerOverflow=on  OutDataTypeStr=Inherit: Same as input  ParamDataTypeStr=Inherit: Same as input
  Complex to Real-Imag : ComplexToRealImag
  Fundamental (PLL-Driven) : spsFundamentalPLLDrivenLib/Fundamental (PLL-Driven)  Finit=50  Fmin=45  InInit=[1, 0]  Ts=Ts_Control
      settings: LibrarySourceBlock=|
      | sps_lib/Sensors and Measurements/Fundamental
      | (PLL-Driven)
  Magnitude-Angle to Complex : MagnitudeAngleToComplex
  Mean : spsMeanLib/Mean  Freq=50  Vinit=415  Ts=Ts_Control
  Mux : Mux  Inputs=2
  PLL : spsPLLLib/PLL  Fmin=45  Par_Init=[0, 50]  ParK=[180, 3200, 1]  TcD=1e-4  MaxRateChangeFreq=12  FilterCutOffFreq=25  Ts=Ts_Control  AGC=on
      settings: LibrarySourceBlock=sps_lib/Control/PLL
  Second-Order Filter : spsSecondOrderFilterLib/Second-Order Filter  FilterType=Lowpass  Fo=2000  Zeta=1  Ts=Ts_Control  Initialize=on  Vac_Init="[0,  0,  60;0,0,60]"  Vdc_Init=[0.9 0]  PlotResponse=off  FreqRange=[0, 500, 1]
      settings: LibrarySourceBlock=|
      | sps_lib/Control/Filters/Second-Order
      | Filter
  Single-Phase dq Transform : Subsystem
  V->pu : Gain  Gain=1/(Vnom_prim*sqrt(2))  SaturateOnIntegerOverflow=on  OutDataTypeStr=Inherit: Same as input  ParamDataTypeStr=Inherit: Same as input
  to-rad : Gain  Gain=pi/180
  Vdc_mean : Outport  VectorParamsAs1DForOutWhenUnconnected=off
  VdVq : Outport  Port=2  VectorParamsAs1DForOutWhenUnconnected=off
  IdIq : Outport  Port=3  VectorParamsAs1DForOutWhenUnconnected=off
  wt : Outport  Port=4  VectorParamsAs1DForOutWhenUnconnected=off
  tag scope: IdIq1=global, Vdc_mean1=global
  wires:
  Mean/1 -> Vdc_mean/1, [Vdc_mean1]
  Vdc/1 -> Mean/1
  to-rad/1 -> Magnitude-Angle to Complex/2
  Mux/1 -> VdVq/1
  Complex to Real-Imag/2 -> Mux/2
  Complex to Real-Imag/1 -> Mux/1
  Magnitude-Angle to Complex/1 -> Complex to Real-Imag/1
  Fundamental (PLL-Driven)/2 -> to-rad/1
  Fundamental (PLL-Driven)/1 -> Magnitude-Angle to Complex/1
  A->pu/1 -> Single-Phase dq Transform/1(Imeas)
  PLL/1 -> Single-Phase dq Transform/3(Freq), Fundamental (PLL-Driven)/1
  PLL/2 -> wt/1, Fundamental (PLL-Driven)/2, Single-Phase dq Transform/2(wt)
  Ihome/1 -> A->pu/1
  Vhome/1 -> V->pu/1
  V->pu/1 -> Fundamental (PLL-Driven)/3, PLL/1
  Single-Phase dq Transform/1(Idq) -> Second-Order Filter/1
  Second-Order Filter/1 -> [IdIq1], IdIq/1

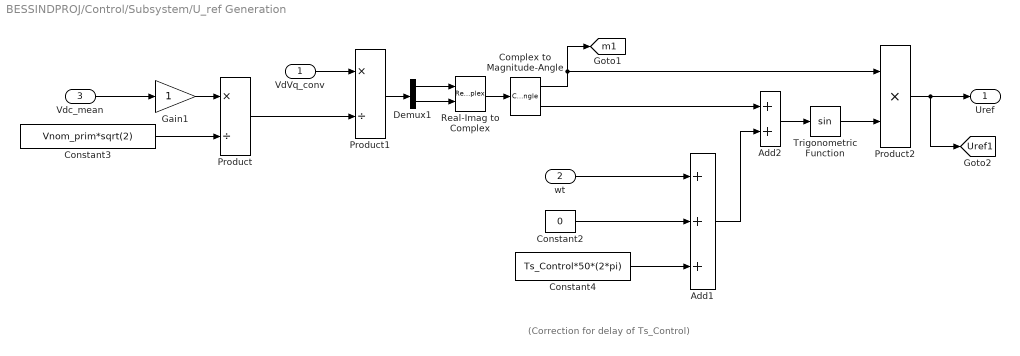
== system BESSINDPROJ/Control/Subsystem/U_ref Generation  ==
  note: (Correction for delay of Ts_Control)
  VdVq_conv : Inport
  wt : Inport  Port=2
  Vdc_mean : Inport  Port=3
  Add1 : Sum  Inputs=+++
  Add2 : Sum
  Complex to Magnitude-Angle : ComplexToMagnitudeAngle
  Constant2 : Constant  Value=0
  Constant3 : Constant  Value=Vnom_prim*sqrt(2)
  Constant4 : Constant  Value=Ts_Control*50*(2*pi)
  Demux1 : Demux  Outputs=2
  Gain1 : Gain
  Product : Product  Inputs=*/  RndMeth=Zero
  Product1 : Product  Inputs=*/  RndMeth=Zero
  Product2 : Product  Inputs=**  RndMeth=Zero
  Real-Imag to Complex : RealImagToComplex
  Trigonometric Function : Trigonometry
  Uref : Outport  VectorParamsAs1DForOutWhenUnconnected=off
  tag scope: Uref1=global, m1=global
  wires:
  VdVq_conv/1 -> Product1/1
  Product2/1 -> Uref/1, [Uref1]
  Vdc_mean/1 -> Gain1/1
  Constant4/1 -> Add1/3
  wt/1 -> Add1/1
  Trigonometric Function/1 -> Product2/2
  Complex to Magnitude-Angle/1 -> [m1], Product2/1
  Add2/1 -> Trigonometric Function/1
  Add1/1 -> Add2/2
  Complex to Magnitude-Angle/2 -> Add2/1
  Product/1 -> Product1/2
  Constant3/1 -> Product/2
  Constant2/1 -> Add1/2
  Demux1/2 -> Real-Imag to Complex/2
  Demux1/1 -> Real-Imag to Complex/1
  Real-Imag to Complex/1 -> Complex to Magnitude-Angle/1
  Gain1/1 -> Product/1
  Product1/1 -> Demux1/1

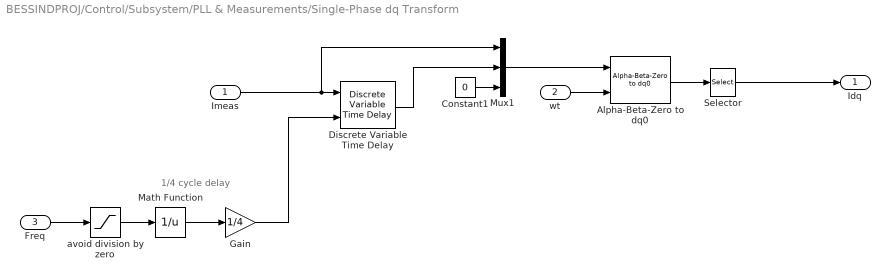
== system BESSINDPROJ/Control/Subsystem/PLL & Measurements/Single-Phase dq Transform ==
  note: 1/4 cycle delay
  Imeas : Inport
  wt : Inport  Port=2
  Freq : Inport  Port=3
  Alpha-Beta-Zero to dq0 : spsAlphaBetaZerotodq0Lib/Alpha-Beta-Zero to dq0  Alignment=90 degrees behind phase A axis
  Constant1 : Constant  Value=0
  Discrete Variable Time Delay : spsDiscreteVariableTimeDelayLib/Discrete Variable Time Delay  MaxDelay=1  InitialValue=0  Ts=Ts_Control  DFT=on
      settings: LibrarySourceBlock=|
      | sps_lib/Control/Discrete Variable
      | Time Delay
  Gain : Gain  Gain=1/4
  Math Function : Math  Operator=reciprocal  SignedPower=on
  Mux1 : Mux  Inputs=3
  Selector : Selector  InputPortWidth=3  IndexOptions=Index vector (dialog)  Indices=[1 2]  OutputSizes=1
  avoid division by zero : Saturate  UpperLimit=70  LowerLimit=40
  Idq : Outport  VectorParamsAs1DForOutWhenUnconnected=off
  wires:
  Constant1/1 -> Mux1/3
  Discrete Variable Time Delay/1 -> Mux1/2
  Mux1/1 -> Alpha-Beta-Zero to dq0/1
  Imeas/1 -> Discrete Variable Time Delay/1, Mux1/1
  wt/1 -> Alpha-Beta-Zero to dq0/2
  Alpha-Beta-Zero to dq0/1 -> Selector/1
  Freq/1 -> avoid division by zero/1
  avoid division by zero/1 -> Math Function/1
  Math Function/1 -> Gain/1
  Gain/1 -> Discrete Variable Time Delay/2
  Selector/1 -> Idq/1

== stateflow chart BESSINDPROJ/Control/Control of Battery ==
  state Battery_Control
    state Entry
    state Surplus_Power
      du:
      state Charge_Battery
        du:
        P_ref=P_load_total;
      state Export_to_grid
        du:
        P_ref=P_pv_total;
      (default) -> Charge_Battery
      Charge_Battery -> Export_to_grid : [Soc_bat>Soc_max]
      Export_to_grid -> Charge_Battery : [Soc_bat<Soc_max]
    state Deficit_Power
      state Discharge_bat
        du:
        P_ref=P_load_total;
      state Import_from_grid
        du:
        P_ref=P_pv_total;
      (default) -> Discharge_bat
      Import_from_grid -> Discharge_bat : [Soc_bat>Soc_min]
      Discharge_bat -> Import_from_grid : [Soc_bat<Soc_critical]
    (default) -> Entry
    Entry -> Surplus_Power [order 1] : [P_pv_total>P_load_total]
    Entry -> Deficit_Power [order 2] : [P_pv_total<P_load_total]
    Surplus_Power -> Deficit_Power : [P_pv_total<P_load_total]
    Deficit_Power -> Surplus_Power : [P_pv_total>P_load_total]
  (default) -> Battery_Control
  data: P_pv_total input; P_load_total input; Soc_bat input; Soc_critical constant double =25; Soc_min constant double =30; Soc_max constant double =90; P_ref output

== matlab function BESSINDPROJ/Control/Subsystem/MPPT Controller using Perturbe & Observe technique  ==
  settings: updateMethod=DISCRETE  sampleTime=Ts_Control
  data: V input; I input; D output
function D  = PandO(  V, I)

% MPPT controller based on the Perturb & Observe algorithm.

% D output = Reference for DC link voltage (Vdc_ref) 
%
% Enabled input = 1 to enable the MPPT controller
% V input = PV array terminal voltage (V)
% I input = PV array current (A)
%
% Param input:
Dinit = 260;  %Initial value for Vdc_ref
Dmax = 290;   %Maximum value for Vdc_ref
Dmin = 230;   %Minimum value for Vdc_ref
deltaD = 0.03; %Increment value used to increase/decrease Vdc_ref
%  

persistent Vold Pold Dold;

dataType = 'double';

if isempty(Vold)
    Vold=0;
    Pold=0;
    Dold=Dinit;
end
P= V*I;
dV= V - Vold;
dP= P - Pold;






if dP ~= 0 
    if dP < 0
        if dV < 0
            D = Dold + deltaD;
        else
            D = Dold - deltaD;
        end
    else
        if dV < 0
            D = Dold - deltaD;
        else
            D = Dold + deltaD;
        end    
    end
else D=Dold;
end

if D >= Dmax | D<= Dmin
    D=Dold;
end

Dold=D;
Vold=V;
Pold=P;
